simulink model "gm_sampleModel1567_1_sub"  (R2023a)
settings: Solver=VariableStepAuto  StartTime=0.0  StopTime=10.0  RelTol=1e-3
libraries: hdlsllib x3
settings Model: Creator=user1  LastModifiedBy=user1
settings OptimizationCC: BlockReduction=off  ConditionallyExecuteInputs=off
settings DebuggingCC: InheritedTsInSrcMsg=none

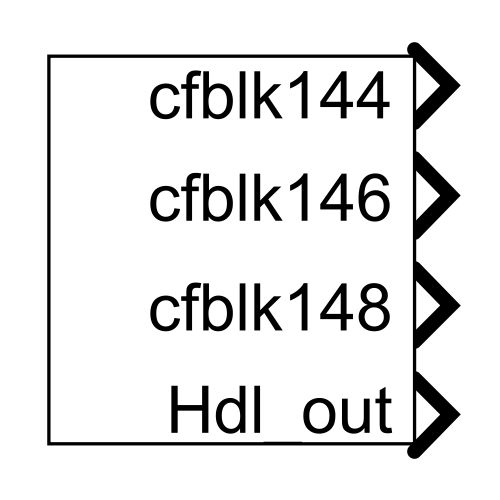
[thumbnail: Simulink's stored preview of the top-level diagram]
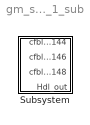
== system gm_sampleModel1567_1_sub ==
  Subsystem : Subsystem

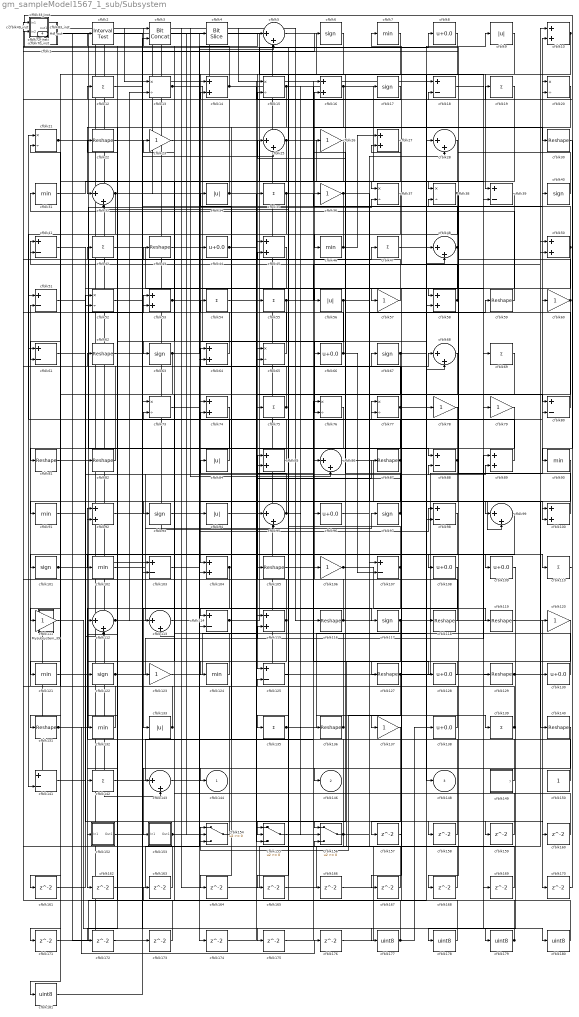
== system gm_sampleModel1567_1_sub/Subsystem ==
  Mysubsystem_39 : Subsystem
  cfblk1 : Subsystem  mask(Detect Rise Positive){vinit=double(0), InputProcessing=Elements as channels (sample based), OutDataTypeStr=uint8}
      mask prompts: vinit "Simulink:masks:InitialCondition_MP"; InputProcessing "Simulink:masks:InputProcessing_MP"; OutDataTypeStr "Simulink:masks:OutputDataType_MP"
      mask help: Simulink:masks:DetectRisePositive_MD
      mask init:
      | InputProcessing = 'Elements as channels (sample based)';
      | OutDataTypeStr = 'uint8';
      | vinit = double(0);
      mask TypeOptions InputProcessing: Simulink:masks:ColumnsAsChannelsFrameBased | Simulink:masks:ElementsAsChannelsSampleBased
      mask TypeOptions OutDataTypeStr: Simulink:masks:uint8 | Simulink:masks:boolean
      mask Display: fprintf('U > 0\n&  NOT\nU/z > 0')
  cfblk{10,14,16,27,45,50,53,58,64,74,85,89,92,100,104,115} (16 alike) : Sum  OutDataTypeStr=uint8
  cfblk{6,17,40,63,67,93,97,101,117,122} (10 alike) : Signum
  cfblk{7,31,46,90..91,102,121,124,132} (9 alike) : MinMax  OutDataTypeStr=uint8
  cfblk{18,39,41,51,61,80,88,98,103,107,114,125,141} (13 alike) : Sum  Inputs=+-  OutDataTypeStr=uint8
  cfblk{22,30,43,59,62,81..82,87,105,116,118..119,127,129,131,136,140} (17 alike) : Reshape
  cfblk{23,26,36,57,60,78..79,106,111,120,123,137} (12 alike) : Gain  OutDataTypeStr=uint8
  cfblk{8,44,66,96,108..109,128,130,138} (9 alike) : Bias  Bias=0.0  SaturateOnIntegerOverflow=off
  cfblk{12,19,35,42,47,54..55,69,75,110,135,139,142} (13 alike) : Sum  Inputs=+  OutDataTypeStr=uint8
  cfblk{5,25,28,32,48,68,86,95,99,112..113,143} (12 alike) : Sum  Inputs=|++  OutDataTypeStr=uint8
  cfblk11_inst : Subsystem
  cfblk126_inst : Subsystem
  cfblk{13,15,20..21,37..38,52,65,73,76..77} (11 alike) : Product  Inputs=*/  OutDataTypeStr=uint8  RndMeth=Zero  SaturateOnIntegerOverflow=on
  cfblk{9,34,56,84,94,133} (6 alike) : Abs  OutDataTypeStr=uint8  SaturateOnIntegerOverflow=off
  cfblk134_inst : Subsystem
  cfblk149 : Subsystem  mask(Counter Free-Running){NumBits=double(16), tsamp=double(-1)}
      mask prompts: NumBits "Simulink:masks:NumberOfBits_MP"; tsamp "Simulink:masks:SampleTime_MP"
      mask help: Simulink:masks:CounterFreeRunning_MD
  cfblk150 : Constant  OutDataTypeStr=uint8  SampleTime=-1
  cfblk152 : Subsystem
  cfblk153 : Subsystem
  cfblk154 : Switch  OutDataTypeStr=uint8  SaturateOnIntegerOverflow=off  InputSameDT=off
  cfblk155 : Switch  OutDataTypeStr=uint8  SaturateOnIntegerOverflow=off  InputSameDT=off
  cfblk156 : Switch  OutDataTypeStr=uint8  SaturateOnIntegerOverflow=off  InputSameDT=off
  cfblk{157..176} (20 alike) : Delay  SampleTime=1
  cfblk{177..181} (5 alike) : DataTypeConversion  OutDataTypeStr=uint8  SaturateOnIntegerOverflow=off  RndMeth=Floor
  cfblk2 : hdlsllib/Logic and Bit Operations/Interval Test  IntervalClosedRight=on  uplimit=0.5  IntervalClosedLeft=on  lowlimit=-0.5  OutDataTypeStr=uint8
  cfblk24_inst : Subsystem
  cfblk29_inst : Subsystem
  cfblk3 : hdlsllib/Logic and Bit Operations/Bit Concat  numInputs=2
  cfblk33_inst : Subsystem
  cfblk4 : hdlsllib/Logic and Bit Operations/Bit Slice  lidx=7  ridx=0
  cfblk49_inst : Subsystem
  cfblk70_inst : Subsystem
  cfblk72_inst : Subsystem
  cfblk83_inst : Subsystem
  cfblk144 : Outport  OutDataTypeStr=uint8  SampleTime=1  VectorParamsAs1DForOutWhenUnconnected=off
  cfblk146 : Outport  Port=2  OutDataTypeStr=uint8  SampleTime=1  VectorParamsAs1DForOutWhenUnconnected=off
  cfblk148 : Outport  Port=3  OutDataTypeStr=uint8  SampleTime=1  VectorParamsAs1DForOutWhenUnconnected=off
  Hdl_out : Outport  Port=4  OutDataTypeStr=uint8  SampleTime=1
  wires:
  Mysubsystem_39/1(Out1) -> cfblk141/1
  cfblk1/1(Y) -> cfblk88/1
  cfblk10/1 -> cfblk39/1, cfblk125/1, cfblk104/1
  cfblk100/1 -> cfblk38/2
  cfblk101/1 -> cfblk77/1, cfblk37/2
  cfblk102/1 -> cfblk97/1
  cfblk103/1 -> cfblk68/1
  cfblk104/1 -> cfblk113/2, cfblk162/1
  cfblk105/1 -> cfblk116/1
  cfblk106/1 -> cfblk155/2, cfblk119/1
  cfblk107/1 -> cfblk32/2, cfblk133/1, cfblk11_inst/2(in2)
  cfblk108/1 -> cfblk156/1
  cfblk109/1 -> cfblk178/1
  cfblk11_inst/1(out1) -> cfblk14/1
  cfblk110/1 -> cfblk49_inst/1(in1)
  cfblk111/1 -> cfblk175/1
  cfblk112/1 -> cfblk89/2, cfblk13/2
  cfblk113/1 -> cfblk74/1
  cfblk114/1 -> cfblk8/1, cfblk19/1
  cfblk115/1 -> cfblk29_inst/1(in1), cfblk152/1(In1)
  cfblk116/1 -> cfblk64/1, cfblk16/2
  cfblk117/1 -> cfblk156/3, cfblk10/2
  cfblk118/1 -> cfblk85/1
  cfblk119/1 -> cfblk170/1
  cfblk12/1 -> cfblk113/1
  cfblk120/1 -> cfblk155/1
  cfblk121/1 -> cfblk53/1
  cfblk122/1 -> cfblk89/1, cfblk45/1, cfblk115/2
  cfblk123/1 -> cfblk115/1
  cfblk124/1 -> cfblk126_inst/1(in1)
  cfblk125/1 -> cfblk15/2
  cfblk126_inst/1(out1) -> cfblk95/2, cfblk35/1
  cfblk127/1 -> cfblk154/1, cfblk60/1
  cfblk128/1 -> cfblk127/1
  cfblk129/1 -> cfblk130/1, Hdl_out/1
  cfblk13/1 -> cfblk118/1, cfblk76/2
  cfblk130/1 -> cfblk42/1
  cfblk131/1 -> cfblk176/1, cfblk47/1
  cfblk132/1 -> cfblk24_inst/1(in1)
  cfblk133/1 -> cfblk92/1, cfblk51/2
  cfblk134_inst/1(out1) -> cfblk18/1
  cfblk135/1 -> cfblk68/2, cfblk139/1
  cfblk136/1 -> cfblk72_inst/1(in1), cfblk11_inst/1(in1)
  cfblk137/1 -> cfblk157/1
  cfblk138/1 -> cfblk23/1
  cfblk139/1 -> cfblk34/1, cfblk21/2
  cfblk14/1 -> cfblk18/2, cfblk134_inst/2(in2)
  cfblk140/1 -> cfblk153/1(In1)
  cfblk141/1 -> cfblk52/1
  cfblk142/1 -> cfblk96/1
  cfblk143/1 -> cfblk174/1
  cfblk149/1(y) -> cfblk54/1
  cfblk15/1 -> cfblk39/2, cfblk32/1, cfblk30/1, cfblk106/1, cfblk124/1
  cfblk150/1 -> cfblk74/2
  cfblk152/1(Out1) -> cfblk25/2
  cfblk153/1(Out1) -> cfblk98/1, cfblk4/1
  cfblk154/1 -> cfblk62/1
  cfblk155/1 -> cfblk159/1
  cfblk156/1 -> cfblk92/2, cfblk59/1, cfblk154/3
  cfblk157/1 -> cfblk77/2
  cfblk158/1 -> cfblk76/1
  cfblk159/1 -> cfblk51/1
  cfblk16/1 -> cfblk53/2, cfblk78/1, cfblk148/1
  cfblk160/1 -> cfblk13/1
  cfblk161/1 -> cfblk88/2
  cfblk162/1 -> cfblk114/2
  cfblk163/1 -> cfblk126_inst/2(in2)
  cfblk164/1 -> cfblk10/1
  cfblk165/1 -> cfblk107/1
  cfblk166/1 -> cfblk28/1
  cfblk167/1 -> cfblk125/2
  cfblk168/1 -> cfblk112/1
  cfblk169/1 -> cfblk15/1
  cfblk17/1 -> cfblk14/2
  cfblk170/1 -> cfblk20/1
  cfblk171/1 -> cfblk48/2
  cfblk172/1 -> cfblk1/1(U)
  cfblk173/1 -> cfblk24_inst/2(in2)
  cfblk174/1 -> cfblk86/1
  cfblk175/1 -> cfblk80/2
  cfblk176/1 -> cfblk50/2
  cfblk177/1 -> cfblk45/2, cfblk138/1, cfblk73/2
  cfblk178/1 -> cfblk2/1
  cfblk179/1 -> cfblk67/1, cfblk163/1
  cfblk18/1 -> cfblk180/1
  cfblk180/1 -> cfblk3/1
  cfblk181/1 -> cfblk3/2
  cfblk19/1 -> cfblk146/1
  cfblk2/1 -> cfblk177/1
  cfblk20/1 -> cfblk132/1
  cfblk21/1 -> cfblk129/1, cfblk103/2
  cfblk22/1 -> cfblk117/1
  cfblk23/1 -> cfblk169/1
  cfblk24_inst/1(out1) -> cfblk86/2, cfblk103/1
  cfblk25/1 -> cfblk37/1, cfblk171/1
  cfblk26/1 -> cfblk63/1
  cfblk27/1 -> cfblk105/1
  cfblk28/1 -> cfblk75/1
  cfblk29_inst/1(out1) -> cfblk143/2, cfblk36/1, cfblk173/1
  cfblk3/1 -> cfblk179/1
  cfblk30/1 -> cfblk90/1
  cfblk31/1 -> cfblk38/1
  cfblk32/1 -> cfblk61/2, cfblk100/2, cfblk100/1
  cfblk33_inst/1(out1) -> cfblk17/1
  cfblk34/1 -> cfblk83_inst/2(in2), cfblk158/1
  cfblk35/1 -> cfblk141/2, cfblk128/1
  cfblk36/1 -> cfblk98/2, cfblk172/1
  cfblk37/1 -> cfblk95/1
  cfblk38/1 -> cfblk168/1, cfblk91/1
  cfblk39/1 -> cfblk57/1
  cfblk4/1 -> cfblk48/1
  cfblk40/1 -> cfblk33_inst/1(in1)
  cfblk41/1 -> cfblk110/1
  cfblk42/1 -> cfblk69/1
  cfblk43/1 -> cfblk56/1
  cfblk44/1 -> cfblk99/2, cfblk80/1
  cfblk45/1 -> cfblk52/2
  cfblk46/1 -> cfblk44/1, cfblk27/1
  cfblk47/1 -> cfblk9/1
  cfblk48/1 -> cfblk16/1, cfblk137/1, cfblk55/1
  cfblk49_inst/1(out1) -> cfblk166/1
  cfblk5/1 -> cfblk79/1
  cfblk50/1 -> cfblk94/1, cfblk27/2
  cfblk51/1 -> cfblk112/2
  cfblk52/1 -> cfblk73/1
  cfblk53/1 -> cfblk66/1, cfblk5/2
  cfblk54/1 -> cfblk108/1
  cfblk55/1 -> cfblk50/1, cfblk136/1, cfblk65/2
  cfblk56/1 -> cfblk58/1, cfblk142/1
  cfblk57/1 -> cfblk70_inst/1(in1)
  cfblk58/1 -> cfblk41/1, cfblk7/1
  cfblk59/1 -> cfblk31/1
  cfblk6/1 -> cfblk64/2
  cfblk60/1 -> cfblk49_inst/2(in2), cfblk167/1
  cfblk61/1 -> cfblk154/2
  cfblk62/1 -> cfblk6/1
  cfblk63/1 -> cfblk5/1, cfblk131/1
  cfblk64/1 -> cfblk33_inst/2(in2)
  cfblk65/1 -> cfblk83_inst/1(in1)
  cfblk66/1 -> cfblk70_inst/2(in2), cfblk107/2
  cfblk67/1 -> cfblk58/2, cfblk155/3, cfblk164/1
  cfblk68/1 -> cfblk111/1
  cfblk69/1 -> cfblk93/1
  cfblk7/1 -> cfblk165/1
  cfblk70_inst/1(out1) -> cfblk29_inst/2(in2), cfblk134_inst/1(in1)
  cfblk72_inst/1(out1) -> cfblk143/1
  cfblk73/1 -> cfblk160/1
  cfblk74/1 -> cfblk161/1
  cfblk75/1 -> cfblk41/2, cfblk22/1
  cfblk76/1 -> cfblk135/1
  cfblk77/1 -> cfblk21/1, cfblk20/2, cfblk102/1
  cfblk78/1 -> cfblk104/2
  cfblk79/1 -> cfblk144/1
  cfblk8/1 -> cfblk46/1
  cfblk80/1 -> cfblk26/1
  cfblk81/1 -> cfblk82/1
  cfblk82/1 -> cfblk72_inst/2(in2)
  cfblk83_inst/1(out1) -> cfblk120/1
  cfblk84/1 -> cfblk61/1
  cfblk85/1 -> cfblk65/1
  cfblk86/1 -> cfblk140/1
  cfblk87/1 -> cfblk114/1, cfblk12/1
  cfblk88/1 -> cfblk81/1, cfblk101/1
  cfblk89/1 -> cfblk43/1
  cfblk9/1 -> cfblk121/1
  cfblk90/1 -> cfblk123/1
  cfblk91/1 -> cfblk109/1
  cfblk92/1 -> cfblk40/1
  cfblk93/1 -> cfblk99/1
  cfblk94/1 -> cfblk87/1
  cfblk95/1 -> cfblk84/1, cfblk156/2
  cfblk96/1 -> cfblk28/2
  cfblk97/1 -> cfblk85/2, cfblk25/1
  cfblk98/1 -> cfblk181/1
  cfblk99/1 -> cfblk122/1

== system gm_sampleModel1567_1_sub/Subsystem/Mysubsystem_39 ==
  cfblk151 : Subsystem  mask(Counter Free-Running){NumBits=double(16), tsamp=double(-1)}
      mask prompts: NumBits "Simulink:masks:NumberOfBits_MP"; tsamp "Simulink:masks:SampleTime_MP"
      mask help: Simulink:masks:CounterFreeRunning_MD
  cfblk71 : Bias  Bias=0.0  SaturateOnIntegerOverflow=off
  Out1 : Outport  SampleTime=1
  wires:
  cfblk151/1(y) -> cfblk71/1
  cfblk71/1 -> Out1/1

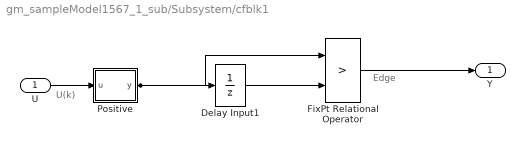
== system gm_sampleModel1567_1_sub/Subsystem/cfblk1 ==
  note: U(k)
  note: Edge
  U : Inport  OutDataTypeStr=uint8  SampleTime=1
  Delay Input1 : UnitDelay  Description=Store in Global RAM  DisableCoverage=on  InitialCondition=vinit  SampleTime=-1  HasFrameUpgradeWarning=on
  FixPt Relational Operator : RelationalOperator  Operator=>  OutDataTypeStr=fixdt(0, 8)  ZeroCross=off  InputSameDT=off
  Positive : Subsystem  mask(Compare To Zero){relop=>, OutDataTypeStr=boolean, ZeroCross=off}
      mask prompts: relop "Simulink:masks:Operator_MP"; OutDataTypeStr "Simulink:masks:OutputDataType_MP"; ZeroCross "Simulink:masks:EnableZerocrossingDetection_MP"
      mask help: Simulink:masks:CompareToZero_MD
      mask init:
      | OutDataTypeStr = 'boolean';
      | ZeroCross = 'off';
      | blkName = 'sampleModel1567_1_sub/Subsystem/cfblk1/Positive';
      | relop = '>';
      | setValue = 'boolean';
      mask TypeOptions relop: == | ~= | < | <= | >= | >
      mask TypeOptions OutDataTypeStr: Simulink:masks:uint8 | Simulink:masks:boolean
      mask Callback ZeroCross: sl('zeroCrossEnable', gcbh);
      mask Display: disp([relop,' 0'])
  Y : Outport  SampleTime=1
  wires:
  U/1 -> Positive/1(u)
  Delay Input1/1 -> FixPt Relational Operator/2
  FixPt Relational Operator/1 -> Y/1
  Positive/1(y) -> FixPt Relational Operator/1, Delay Input1/1

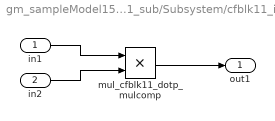
== system gm_sampleModel1567_1_sub/Subsystem/cfblk11_inst ==
  in1 : Inport  OutDataTypeStr=uint8  SampleTime=1
  in2 : Inport  Port=2  OutDataTypeStr=uint8  SampleTime=1
  mul_cfblk11_dotp_mulcomp : Product  Inputs=**  OutDataTypeStr=uint8  SampleTime=1
  out1 : Outport  OutDataTypeStr=uint8  SampleTime=1
  wires:
  in1/1 -> mul_cfblk11_dotp_mulcomp/1
  in2/1 -> mul_cfblk11_dotp_mulcomp/2
  mul_cfblk11_dotp_mulcomp/1 -> out1/1

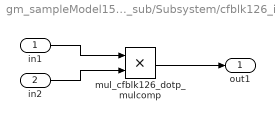
== system gm_sampleModel1567_1_sub/Subsystem/cfblk126_inst ==
  in1 : Inport  OutDataTypeStr=uint8  SampleTime=1
  in2 : Inport  Port=2  OutDataTypeStr=uint8  SampleTime=1
  mul_cfblk126_dotp_mulcomp : Product  Inputs=**  OutDataTypeStr=uint8  SampleTime=1
  out1 : Outport  OutDataTypeStr=uint8  SampleTime=1
  wires:
  in1/1 -> mul_cfblk126_dotp_mulcomp/1
  in2/1 -> mul_cfblk126_dotp_mulcomp/2
  mul_cfblk126_dotp_mulcomp/1 -> out1/1

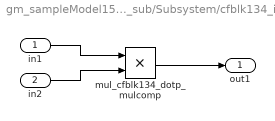
== system gm_sampleModel1567_1_sub/Subsystem/cfblk134_inst ==
  in1 : Inport  OutDataTypeStr=uint8  SampleTime=1
  in2 : Inport  Port=2  OutDataTypeStr=uint8  SampleTime=1
  mul_cfblk134_dotp_mulcomp : Product  Inputs=**  OutDataTypeStr=uint8  SampleTime=1
  out1 : Outport  OutDataTypeStr=uint8  SampleTime=1
  wires:
  in1/1 -> mul_cfblk134_dotp_mulcomp/1
  in2/1 -> mul_cfblk134_dotp_mulcomp/2
  mul_cfblk134_dotp_mulcomp/1 -> out1/1

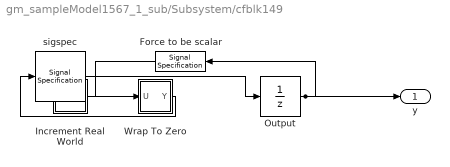
== system gm_sampleModel1567_1_sub/Subsystem/cfblk149 ==
  Force to be scalar : SignalSpecification  DisableCoverage=on  Dimensions=1
  Increment Real World : Subsystem  mask(Real World Value Increment){}
      mask help: Simulink:masks:RealWorldValueIncrement_MD
      mask Display: disp('V++')
  Output : UnitDelay  InitialCondition=0.0  SampleTime=tsamp  HasFrameUpgradeWarning=on
  Wrap To Zero : Subsystem  mask(Wrap To Zero){Threshold=double(65535)}
      mask prompts: Threshold "Simulink:masks:Threshold_MP"
      mask help: Simulink:masks:WrapToZero_MD
  sigspec : SignalSpecification  OutDataTypeStr=uint16  Dimensions=1
  y : Outport  SampleTime=1
  wires:
  Force to be scalar/1 -> Increment Real World/1(u)
  Increment Real World/1(y) -> Wrap To Zero/1(U)
  Output/1 -> Force to be scalar/1, y/1
  Wrap To Zero/1(Y) -> sigspec/1
  sigspec/1 -> Output/1

== system gm_sampleModel1567_1_sub/Subsystem/cfblk152 ==
  In1 : Inport  OutDataTypeStr=uint8  PortDimensions=1  SampleTime=1
  Out1 : Outport  SampleTime=1
  wires:
  In1/1 -> Out1/1

== system gm_sampleModel1567_1_sub/Subsystem/cfblk153 ==
  In1 : Inport  OutDataTypeStr=uint8  PortDimensions=1  SampleTime=1
  Out1 : Outport  SampleTime=1
  wires:
  In1/1 -> Out1/1

== system gm_sampleModel1567_1_sub/Subsystem/cfblk24_inst ==
  in1 : Inport  OutDataTypeStr=uint8  SampleTime=1
  in2 : Inport  Port=2  OutDataTypeStr=uint8  SampleTime=1
  mul_cfblk24_dotp_mulcomp : Product  Inputs=**  OutDataTypeStr=uint8  SampleTime=1
  out1 : Outport  OutDataTypeStr=uint8  SampleTime=1
  wires:
  in1/1 -> mul_cfblk24_dotp_mulcomp/1
  in2/1 -> mul_cfblk24_dotp_mulcomp/2
  mul_cfblk24_dotp_mulcomp/1 -> out1/1

== system gm_sampleModel1567_1_sub/Subsystem/cfblk29_inst ==
  in1 : Inport  OutDataTypeStr=uint8  SampleTime=1
  in2 : Inport  Port=2  OutDataTypeStr=uint8  SampleTime=1
  mul_cfblk29_dotp_mulcomp : Product  Inputs=**  OutDataTypeStr=uint8  SampleTime=1
  out1 : Outport  OutDataTypeStr=uint8  SampleTime=1
  wires:
  in1/1 -> mul_cfblk29_dotp_mulcomp/1
  in2/1 -> mul_cfblk29_dotp_mulcomp/2
  mul_cfblk29_dotp_mulcomp/1 -> out1/1

== system gm_sampleModel1567_1_sub/Subsystem/cfblk33_inst ==
  in1 : Inport  OutDataTypeStr=uint8  SampleTime=1
  in2 : Inport  Port=2  OutDataTypeStr=uint8  SampleTime=1
  mul_cfblk33_dotp_mulcomp : Product  Inputs=**  OutDataTypeStr=uint8  SampleTime=1
  out1 : Outport  OutDataTypeStr=uint8  SampleTime=1
  wires:
  in1/1 -> mul_cfblk33_dotp_mulcomp/1
  in2/1 -> mul_cfblk33_dotp_mulcomp/2
  mul_cfblk33_dotp_mulcomp/1 -> out1/1

== system gm_sampleModel1567_1_sub/Subsystem/cfblk49_inst ==
  in1 : Inport  OutDataTypeStr=uint8  SampleTime=1
  in2 : Inport  Port=2  OutDataTypeStr=uint8  SampleTime=1
  mul_cfblk49_dotp_mulcomp : Product  Inputs=**  OutDataTypeStr=uint8  SampleTime=1
  out1 : Outport  OutDataTypeStr=uint8  SampleTime=1
  wires:
  in1/1 -> mul_cfblk49_dotp_mulcomp/1
  in2/1 -> mul_cfblk49_dotp_mulcomp/2
  mul_cfblk49_dotp_mulcomp/1 -> out1/1

== system gm_sampleModel1567_1_sub/Subsystem/cfblk70_inst ==
  in1 : Inport  OutDataTypeStr=uint8  SampleTime=1
  in2 : Inport  Port=2  OutDataTypeStr=uint8  SampleTime=1
  mul_cfblk70_dotp_mulcomp : Product  Inputs=**  OutDataTypeStr=uint8  SampleTime=1
  out1 : Outport  OutDataTypeStr=uint8  SampleTime=1
  wires:
  in1/1 -> mul_cfblk70_dotp_mulcomp/1
  in2/1 -> mul_cfblk70_dotp_mulcomp/2
  mul_cfblk70_dotp_mulcomp/1 -> out1/1

== system gm_sampleModel1567_1_sub/Subsystem/cfblk72_inst ==
  in1 : Inport  OutDataTypeStr=uint8  SampleTime=1
  in2 : Inport  Port=2  OutDataTypeStr=uint8  SampleTime=1
  mul_cfblk72_dotp_mulcomp : Product  Inputs=**  OutDataTypeStr=uint8  SampleTime=1
  out1 : Outport  OutDataTypeStr=uint8  SampleTime=1
  wires:
  in1/1 -> mul_cfblk72_dotp_mulcomp/1
  in2/1 -> mul_cfblk72_dotp_mulcomp/2
  mul_cfblk72_dotp_mulcomp/1 -> out1/1

== system gm_sampleModel1567_1_sub/Subsystem/cfblk83_inst ==
  in1 : Inport  OutDataTypeStr=uint8  SampleTime=1
  in2 : Inport  Port=2  OutDataTypeStr=uint8  SampleTime=1
  mul_cfblk83_dotp_mulcomp : Product  Inputs=**  OutDataTypeStr=uint8  SampleTime=1
  out1 : Outport  OutDataTypeStr=uint8  SampleTime=1
  wires:
  in1/1 -> mul_cfblk83_dotp_mulcomp/1
  in2/1 -> mul_cfblk83_dotp_mulcomp/2
  mul_cfblk83_dotp_mulcomp/1 -> out1/1

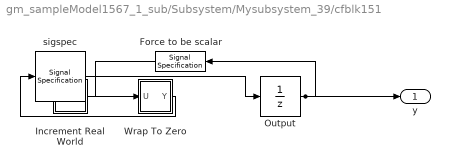
== system gm_sampleModel1567_1_sub/Subsystem/Mysubsystem_39/cfblk151 ==
  Force to be scalar : SignalSpecification  DisableCoverage=on  Dimensions=1
  Increment Real World : Subsystem  mask(Real World Value Increment){}
      mask help: Simulink:masks:RealWorldValueIncrement_MD
      mask Display: disp('V++')
  Output : UnitDelay  InitialCondition=0.0  SampleTime=tsamp  HasFrameUpgradeWarning=on
  Wrap To Zero : Subsystem  mask(Wrap To Zero){Threshold=double(65535)}
      mask prompts: Threshold "Simulink:masks:Threshold_MP"
      mask help: Simulink:masks:WrapToZero_MD
  sigspec : SignalSpecification  OutDataTypeStr=uint16  Dimensions=1
  y : Outport  SampleTime=1
  wires:
  Force to be scalar/1 -> Increment Real World/1(u)
  Increment Real World/1(y) -> Wrap To Zero/1(U)
  Output/1 -> Force to be scalar/1, y/1
  Wrap To Zero/1(Y) -> sigspec/1
  sigspec/1 -> Output/1

== system gm_sampleModel1567_1_sub/Subsystem/cfblk1/Positive ==
  u : Inport  OutDataTypeStr=uint8  SampleTime=1
  Compare : RelationalOperator  Operator=>  OutDataTypeStr=boolean  ZeroCross=off
  Constant : Constant  DisableCoverage=on  Value=0  OutDataTypeStr=Inherit: Inherit via back propagation  SampleTime=-1  PreserveConstantTs=on
  y : Outport  SampleTime=1
  wires:
  u/1 -> Compare/1
  Compare/1 -> y/1
  Constant/1 -> Compare/2

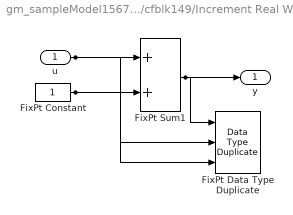
== system gm_sampleModel1567_1_sub/Subsystem/cfblk149/Increment Real World ==
  u : Inport  OutDataTypeStr=uint16  SampleTime=1
  FixPt Constant : Constant  DisableCoverage=on  OutDataTypeStr=Inherit: Inherit via back propagation  SampleTime=-1
  FixPt Data Type Duplicate : DataTypeDuplicate  DisableCoverage=on  NumInputPorts=3
  FixPt Sum1 : Sum  InputSameDT=on  OutDataTypeStr=Inherit: Inherit via back propagation  LockScale=on
  y : Outport  SampleTime=1
  wires:
  u/1 -> FixPt Sum1/1, FixPt Data Type Duplicate/2
  FixPt Constant/1 -> FixPt Sum1/2, FixPt Data Type Duplicate/3
  FixPt Sum1/1 -> FixPt Data Type Duplicate/1, y/1

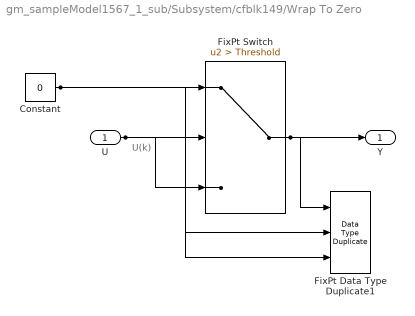
== system gm_sampleModel1567_1_sub/Subsystem/cfblk149/Wrap To Zero ==
  note: U(k)
  U : Inport  OutDataTypeStr=uint16  SampleTime=1
  Constant : Constant  DisableCoverage=on  Value=0  OutDataTypeStr=Inherit: Inherit via back propagation  SampleTime=-1
  FixPt Data Type Duplicate1 : DataTypeDuplicate  DisableCoverage=on  NumInputPorts=3
  FixPt Switch : Switch  Criteria=u2 > Threshold  Threshold=Threshold  OutDataTypeStr=Inherit: Inherit via back propagation  ZeroCross=off  SaturateOnIntegerOverflow=off  InputSameDT=off
  Y : Outport  SampleTime=1
  wires:
  U/1 -> FixPt Switch/3, FixPt Switch/2, FixPt Data Type Duplicate1/2
  Constant/1 -> FixPt Switch/1, FixPt Data Type Duplicate1/3
  FixPt Switch/1 -> FixPt Data Type Duplicate1/1, Y/1

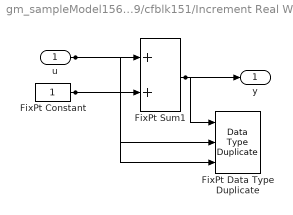
== system gm_sampleModel1567_1_sub/Subsystem/Mysubsystem_39/cfblk151/Increment Real World ==
  u : Inport  OutDataTypeStr=uint16  SampleTime=1
  FixPt Constant : Constant  DisableCoverage=on  OutDataTypeStr=Inherit: Inherit via back propagation  SampleTime=-1
  FixPt Data Type Duplicate : DataTypeDuplicate  DisableCoverage=on  NumInputPorts=3
  FixPt Sum1 : Sum  InputSameDT=on  OutDataTypeStr=Inherit: Inherit via back propagation  LockScale=on
  y : Outport  SampleTime=1
  wires:
  u/1 -> FixPt Sum1/1, FixPt Data Type Duplicate/2
  FixPt Constant/1 -> FixPt Sum1/2, FixPt Data Type Duplicate/3
  FixPt Sum1/1 -> FixPt Data Type Duplicate/1, y/1

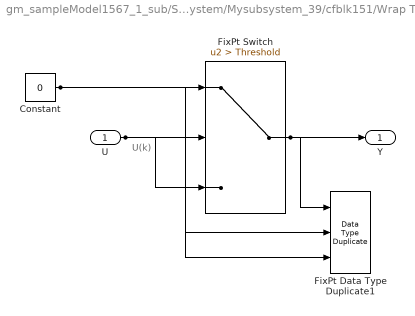
== system gm_sampleModel1567_1_sub/Subsystem/Mysubsystem_39/cfblk151/Wrap To Zero ==
  note: U(k)
  U : Inport  OutDataTypeStr=uint16  SampleTime=1
  Constant : Constant  DisableCoverage=on  Value=0  OutDataTypeStr=Inherit: Inherit via back propagation  SampleTime=-1
  FixPt Data Type Duplicate1 : DataTypeDuplicate  DisableCoverage=on  NumInputPorts=3
  FixPt Switch : Switch  Criteria=u2 > Threshold  Threshold=Threshold  OutDataTypeStr=Inherit: Inherit via back propagation  ZeroCross=off  SaturateOnIntegerOverflow=off  InputSameDT=off
  Y : Outport  SampleTime=1
  wires:
  U/1 -> FixPt Switch/3, FixPt Switch/2, FixPt Data Type Duplicate1/2
  Constant/1 -> FixPt Switch/1, FixPt Data Type Duplicate1/3
  FixPt Switch/1 -> FixPt Data Type Duplicate1/1, Y/1
